simulink model "B_transition"  (R2020a)
settings: Solver=FixedStepDiscrete  StartTime=0.0  StopTime=800  FixedStep=0.1  RelTol=1e-3  EnableMultiTasking=on
settings Model: Creator=hp-pc  LastModifiedBy=hp-pc
settings SolverCC: AutoInsertRateTranBlk=on
settings DataIOCC: LimitDataPoints=on
settings OptimizationCC: LifeSpan=inf
settings DebuggingCC: AllowSymbolicDim=off  SFUnexpectedBacktrackingDiag=warning  SFNoUnconditionalDefaultTransitionDiag=warning  SFExecutionAtInitializationDiag=none  ArithmeticOperatorsInVariantConditions=warning
settings SFSimCC: SimUseLocalCustomCode=off  CustomCodeUndefinedFunction=UseInterfaceOnly
settings RTWCC: RTWUseLocalCustomCode=off
settings CodeAppCC: StateflowObjectComments=on
settings GRTTargetCC: TargetLangStandard=C89/C90 (ANSI)
settings ConfigComp: CovMetricSettings=dw  CovHtmlReporting=on  CovSaveCumulativeToWorkspaceVar=on  CovSaveSingleToWorkspaceVar=on  CovShowResultsExplorer=off  CovExternalEMLEnable=off  CovSFcnEnable=off

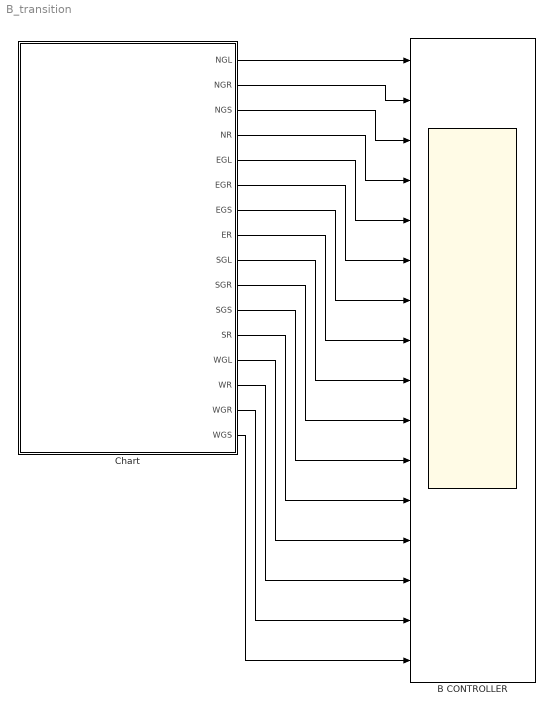
== system B_transition ==
  B CONTROLLER : Scope  NumInputPorts=16
  Chart : Stateflow chart  TreatAsAtomicUnit=on
  wires:
  Chart/2(NGR) -> B CONTROLLER/2
  Chart/4(NR) -> B CONTROLLER/4
  Chart/5(EGL) -> B CONTROLLER/5
  Chart/13(WGL) -> B CONTROLLER/13
  Chart/10(SGR) -> B CONTROLLER/10
  Chart/15(WGR) -> B CONTROLLER/15
  Chart/6(EGR) -> B CONTROLLER/6
  Chart/11(SGS) -> B CONTROLLER/11
  Chart/12(SR) -> B CONTROLLER/12
  Chart/14(WR) -> B CONTROLLER/14
  Chart/16(WGS) -> B CONTROLLER/16
  Chart/3(NGS) -> B CONTROLLER/3
  Chart/7(EGS) -> B CONTROLLER/7
  Chart/1(NGL) -> B CONTROLLER/1
  Chart/9(SGL) -> B CONTROLLER/9
  Chart/8(ER) -> B CONTROLLER/8

== stateflow chart B_transition/Chart ==
  state B1
    state NB [parallel]
      NGS=1;NGL=1;NGR=1;
      NR=0;
      settings: executionOrder=1
    state SB [parallel]
      SGS=0;SGL=0;SGR=0;
      SR=1;
      settings: executionOrder=2
    state EB [parallel]
      EGS=0;EGL=0;EGR=0;
      ER=1;
      settings: executionOrder=3
    state WB [parallel]
      WGS=0;WGL=0;WGR=0;
      WR=1;
      settings: executionOrder=4
  state B2
    state NB [parallel]
      NGS=1;NGL=0;NGR=1;
      NR=0;
      settings: executionOrder=1
    state SB [parallel]
      SGS=1;SGL=0;SGR=1;
      SR=0;
      settings: executionOrder=2
    state EB [parallel]
      EGS=0;EGL=0;EGR=0;
      ER=1;
      settings: executionOrder=3
    state WB [parallel]
      WGS=0;WGL=0;WGR=0;
      WR=1;
      settings: executionOrder=4
  state B3
    state NB [parallel]
      NGS=0;NGL=0;NGR=0;
      NR=1;
      settings: executionOrder=1
    state SB [parallel]
      SGS=1;SGL=1;SGR=1;
      SR=0;
      settings: executionOrder=2
    state EB [parallel]
      EGS=0;EGL=0;EGR=0;
      ER=1;
      settings: executionOrder=3
    state WB [parallel]
      WGS=0;WGL=0;WGR=0;
      WR=1;
      settings: executionOrder=4
  state B6
    state NB [parallel]
      NGS=0;NGL=0;NGR=0;
      NR=1;
      settings: executionOrder=1
    state SB [parallel]
      SGS=0;SGL=0;SGR=0;
      SR=1;
      settings: executionOrder=2
    state EB [parallel]
      EGS=1;EGL=1;EGR=1;
      ER=0;
      settings: executionOrder=3
    state WB [parallel]
      WGS=0;WGL=0;WGR=0;
      WR=1;
      settings: executionOrder=4
  state B5
    state NB [parallel]
      NGS=0;NGL=0;NGR=0;
      NR=1;
      settings: executionOrder=1
    state SB [parallel]
      SGS=0;SGL=0;SGR=0;
      SR=1;
      settings: executionOrder=2
    state EB [parallel]
      EGS=1;EGL=0;EGR=1;
      ER=0;
      settings: executionOrder=3
    state WB [parallel]
      WGS=1;WGL=0;WGR=1;
      WR=0;
      settings: executionOrder=4
  state B4
    state NB [parallel]
      NGS=0;NGL=0;NGR=0;
      NR=1;
      settings: executionOrder=1
    state SB [parallel]
      SGS=0;SGL=0;SGR=0;
      SR=1;
      settings: executionOrder=2
    state EB [parallel]
      EGS=0;EGL=0;EGR=0;
      ER=1;
      settings: executionOrder=3
    state WB [parallel]
      WGS=1;WGL=1;WGR=1;
      WR=0;
      settings: executionOrder=4
  (default) -> B1
  B1 -> B2 : after(45,sec)
  B2 -> B3 : after(90,sec)
  B6 -> B1 : after(90,sec)
  B3 -> B4 : after(90,sec)
  B4 -> B5 : after(45,sec)
  B5 -> B6 : after(90,sec)
  data: NGL output; NGR output; NGS output; NR output; EGL output; EGR output; EGS output; ER output; SGL output; SGR output; SGS output; SR output; WGL output; WR output; WGR output; WGS output
